simulink model "project"  (R2018b)
settings: Solver=FixedStepDiscrete  StartTime=0.0  StopTime=inf  FixedStep=3.1189083820662764e-10  RelTol=1e-3
values from neighbouring files (symbols this model uses):
  espacement_pilote = 4    [matlab.mat]
  N = 10    [matlab.mat]
  N_cyclic = 3    [matlab.mat]
  N_total = 16    [matlab.mat]
  Ts = 5.92592592593e-06    [matlab.mat]
undefined symbols (not defined in the file or in its folder): doppler
libraries: dspxfrm3 x5, commchan3 x2, commdigbbndpm3 x2, commrandsrc3 x1, commsink2 x1, dspfdesign x1
settings Model: SimulationMode=accelerator  Creator=rcalizzano  LastModifiedBy=nijac19
settings SolverCC: AutoInsertRateTranBlk=on
settings DataIOCC: LimitDataPoints=on  SaveOutput=off  SignalLogging=off  SaveTime=off
settings OptimizationCC: LifeSpan=inf
settings DebuggingCC: AlgebraicLoopMsg=error  SingleTaskRateTransMsg=error  AllowSymbolicDim=off  SFUnexpectedBacktrackingDiag=warning  SFNoUnconditionalDefaultTransitionDiag=warning  SFExecutionAtInitializationDiag=none
settings SFSimCC: SimUseLocalCustomCode=off
settings RTWCC: RTWUseLocalCustomCode=off
settings CodeAppCC: StateflowObjectComments=on
settings GRTTargetCC: TargetLangStandard=C89/C90 (ANSI)  GeneratePreprocessorConditionals=Disable all

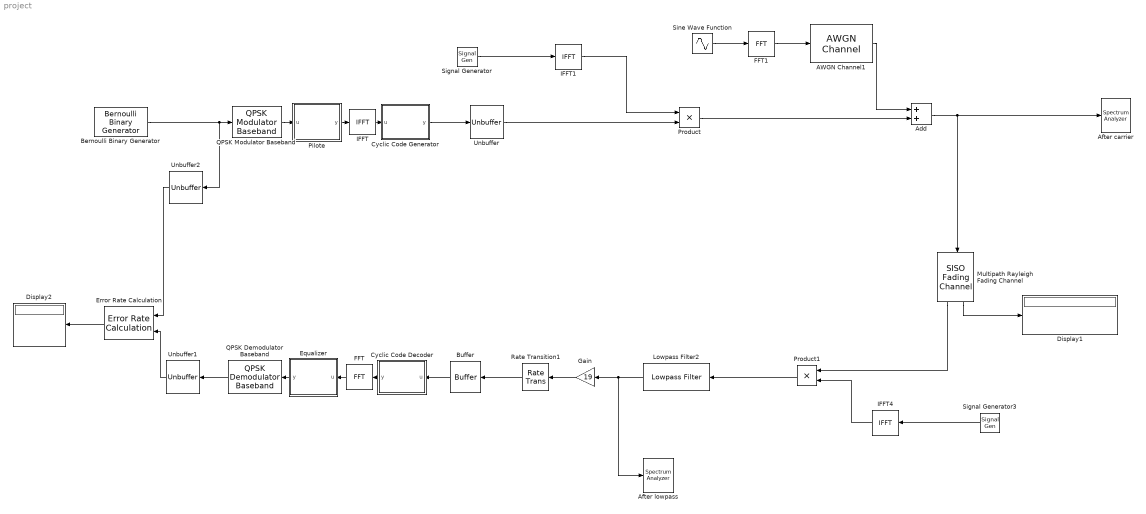
== system project ==
  AWGN Channel1 : commchan3/AWGN Channel  InputProcessing=Columns as channels (frame based)  seed=67  noiseMode="Signal to noise ratio  (SNR)"  EbNodB=10  EsNodB=10  SNRdB=150  bitsPerSym=1  Ps=4e4  Tsym=1  variance=1
  Add : Sum
  "After carrier " : SpectrumAnalyzer
  After lowpass : SpectrumAnalyzer
  Bernoulli Binary Generator : commrandsrc3/Bernoulli Binary Generator  ProbabilityOfZero=0.5  SeedSource=Auto  Seed=0  SampleTime=Ts/(N*2)  SamplesPerFrame=N*2  OutputDataType=double  SimulateUsing=Interpreted execution
      settings: SourceProductName=Communications Toolbox
  Buffer : Buffer  N=N_total+N_cyclic  OutputFrames=off
  Cyclic Code Decoder : MATLAB Function  TreatAsAtomicUnit=on
  Cyclic Code Generator : MATLAB Function  TreatAsAtomicUnit=on
  Display1 : Display
  Display2 : Display
  Equalizer : MATLAB Function  TreatAsAtomicUnit=on
  Error Rate Calculation : commsink2/Error Rate Calculation  N=N*2  st_delay=0  cp_mode=Entire frame  subframe=[]  PMode=Port  WsName=ErrorVec  RsMode2=off  stop=off  numErr=100  maxBits=1e6
      settings: SourceProductName=Communications Toolbox
  FFT : dspxfrm3/FFT  FFTImplementation=Auto  CompMethod=Table lookup  TableOpt=NEW  TableOptActive=Speed  BitRevOrder=off  Normalize=off  InheritFFTLength=on  FFTLength=64  WrapInput=on  roundingMode=Floor  overflowMode=off  firstCoeffDataTypeStr=Inherit: Same word length as input  firstCoeffLastDataTypeStr=Inherit: Same word length as input  outputMin=[]  outputMax=[]
  FFT1 : dspxfrm3/FFT  FFTImplementation=Auto  CompMethod=Table lookup  TableOpt=NEW  TableOptActive=Speed  BitRevOrder=off  Normalize=off  InheritFFTLength=on  FFTLength=64  WrapInput=on  roundingMode=Floor  overflowMode=off  firstCoeffDataTypeStr=Inherit: Same word length as input  firstCoeffLastDataTypeStr=Inherit: Same word length as input  outputMin=[]  outputMax=[]
  Gain : Gain  Gain=19
  IFFT : dspxfrm3/IFFT  FFTImplementation=Auto  CompMethod=Table lookup  TableOpt=NEW  TableOptActive=Speed  BitRevOrder=off  cs_in=off  Normalize=on  InheritFFTLength=on  FFTLength=64  WrapInput=on  mode=Complex  outSamplingMode=Sample based  roundingMode=Floor  overflowMode=off  firstCoeffDataTypeStr=Inherit: Same word length as input  firstCoeffLastDataTypeStr=Inherit: Same word length as input  outputMin=[]  outputMax=[]
      settings: SourceProductName=DSP System Toolbox
  IFFT1 : dspxfrm3/IFFT  FFTImplementation=Auto  CompMethod=Table lookup  TableOpt=NEW  TableOptActive=Speed  BitRevOrder=off  cs_in=off  Normalize=on  InheritFFTLength=on  FFTLength=64  WrapInput=on  mode=Complex  outSamplingMode=Sample based  roundingMode=Floor  overflowMode=off  firstCoeffDataTypeStr=Inherit: Same word length as input  firstCoeffLastDataTypeStr=Inherit: Same word length as input  outputMin=[]  outputMax=[]
      settings: SourceProductName=DSP System Toolbox
  IFFT4 : dspxfrm3/IFFT  FFTImplementation=Auto  CompMethod=Table lookup  TableOpt=NEW  TableOptActive=Speed  BitRevOrder=off  cs_in=off  Normalize=on  InheritFFTLength=on  FFTLength=64  WrapInput=on  mode=Complex  outSamplingMode=Sample based  roundingMode=Floor  overflowMode=off  firstCoeffDataTypeStr=Inherit: Same word length as input  firstCoeffLastDataTypeStr=Inherit: Same word length as input  outputMin=[]  outputMax=[]
      settings: SourceProductName=DSP System Toolbox
  Lowpass Filter2 : dspfdesign/Lowpass Filter  FilterType=IIR  DesignForMinimumOrder=on  FilterOrder=50  PassbandFrequency=fpass  StopbandFrequency=fstop  PassbandRipple=0.1  StopbandAttenuation=180  InheritSampleRate=on  SampleRate=1/15.5945e-009  SimulateUsing=Interpreted execution  roundingMode=Floor  coeffsDataTypeStr=fixdt(1,16)
  Multipath Rayleigh Fading Channel : commchan3/SISO Fading Channel  InheritSampleRate=on  SampleRate=1  PathDelays=[0]  AveragePathGains=[0]  NormalizePathGains=on  FadingDistribution=Rayleigh  KFactor=3  DirectPathDopplerShift=0  DirectPathInitialPhase=0  MaximumDopplerShift=0.01  DopplerSpectrum=doppler('Jakes')  ChannelInterpolationMethod=Polyphase  RandomStream=mt19937ar with seed  RandomNumGenerator=shr3cong  Seed=73  PathGainsOutputPort=on  ChannelFilterDelayOutputPort=off  SimulateUsing=Interpreted execution  Visualization=Off  PathsForDopplerDisplay=1  SamplesToDisplay=25%
      settings: SourceProductName=Communications Toolbox
  Pilote : MATLAB Function  TreatAsAtomicUnit=on
  Product : Product
  Product1 : Product
  QPSK Demodulator Baseband : commdigbbndpm3/QPSK Demodulator Baseband  OutType=Bit  DecType=Hard decision  VarSource=Dialog  Variance=1  Dec=Gray  Ph=pi/4  outDtype1=Inherit via internal rule  outDtype2=Inherit via internal rule  derotateFactorWordLen=16  derotateFactorDataTypeStr=Inherit: Same word length as input  derotateFactorLastDataTypeStr=Inherit: Same word length as input
      settings: SourceProductName=Communications Toolbox
  QPSK Modulator Baseband : commdigbbndpm3/QPSK Modulator Baseband  InType=Bit  Enc=Gray  Ph=pi/4  outDtype=double  outWordLen=16  outUDDataType=sfix(16)  outFracLenMode=Best precision  outFracLen=15  outDataTypeStr=double  outLastDataTypeStr=double
      settings: SourceProductName=Communications Toolbox
  Rate Transition1 : RateTransition
  Signal Generator : SignalGenerator  Amplitude=0.325  Frequency=868e6
  Signal Generator3 : SignalGenerator  Amplitude=0.325  Frequency=868e6
  Sine Wave Function : Sin  Amplitude=4e4  Frequency=314.159265  SampleTime=0
  Unbuffer : Unbuffer
  Unbuffer1 : Unbuffer
  Unbuffer2 : Unbuffer
  wires:
  QPSK Demodulator Baseband/1 -> Unbuffer1/1
  Unbuffer1/1 -> Error Rate Calculation/2
  Error Rate Calculation/1 -> Display2/1
  Unbuffer2/1 -> Error Rate Calculation/1
  Multipath Rayleigh Fading Channel/2 -> Display1/1
  Bernoulli Binary Generator/1 -> QPSK Modulator Baseband/1, Unbuffer2/1
  IFFT/1 -> Cyclic Code Generator/1(u)
  Cyclic Code Decoder/1(y) -> FFT/1
  QPSK Modulator Baseband/1 -> Pilote/1(u)
  Buffer/1 -> Cyclic Code Decoder/1(u)
  Equalizer/1(y) -> QPSK Demodulator Baseband/1
  Pilote/1(y) -> IFFT/1
  Cyclic Code Generator/1(y) -> Unbuffer/1
  FFT/1 -> Equalizer/1(u)
  IFFT1/1 -> Product/1
  Sine Wave Function/1 -> FFT1/1
  FFT1/1 -> AWGN Channel1/1
  Rate Transition1/1 -> Buffer/1
  AWGN Channel1/1 -> Add/1
  Product1/1 -> Lowpass Filter2/1
  Lowpass Filter2/1 -> After lowpass/1, Gain/1
  Signal Generator/1 -> IFFT1/1
  Gain/1 -> Rate Transition1/1
  Unbuffer/1 -> Product/2
  Signal Generator3/1 -> IFFT4/1
  IFFT4/1 -> Product1/2
  Product/1 -> Add/2
  Add/1 -> Multipath Rayleigh Fading Channel/1, "After carrier "/1
  Multipath Rayleigh Fading Channel/1 -> Product1/1

== matlab function project/Cyclic Code Decoder ==
  data: u input; y output; N_cyclic parameter
function y = fcn(u, N_cyclic)

y = u(N_cyclic+1:end);

== matlab function project/Pilote ==
  data: u input; N parameter; y output; N_total parameter; espacement_pilote parameter
function y  = fcn(u, N, N_total, espacement_pilote)

N_pilote = floor(N/espacement_pilote);
N_zeros = N_total-N-N_pilote;

w = complex(zeros(floor(N+N/espacement_pilote),1), zeros(floor(N+N/espacement_pilote),1));

% Insertion des pilotes

compteur = 0;
for i = [1:N]
    if mod(i,espacement_pilote) == espacement_pilote/2+1
        if compteur < N_pilote    
            w(i+compteur) = complex(1,0);
            compteur = compteur +1;
        end
        w(i+compteur) = u(i);
    else
        w(i+compteur) = u(i);
    end
end

% Insertion des zeros

y = [w(1:floor((N+floor(N/espacement_pilote))/2)); complex(zeros(N_zeros,1),zeros(N_zeros,1)); w(floor((N+floor(N/espacement_pilote))/2+1):end)];

== matlab function project/Cyclic Code Generator ==
  data: u input; y output; N_cyclic parameter; N_total parameter
function y = fcn(u, N_cyclic, N_total)

u_end = u(N_total-N_cyclic+1:end);

y = [u_end; u];

== matlab function project/Equalizer ==
  data: u input; y output; N parameter; N_total parameter; espacement_pilote parameter
function y = fcn(u, N, N_total, espacement_pilote)

N_pilote = floor(N/espacement_pilote);
N_zeros = N_total-N-N_pilote;

gain = complex(zeros(N_pilote,1), zeros(N_pilote,1));
gain_plot = complex(zeros(N_pilote+N,1), zeros(N_pilote+N,1));


% On enlève les zeros

w = [u(1:floor((N_total-N_zeros)/2)); u(floor((N_total-N_zeros)/2+N_zeros+1):end)];

% On initialise les valeurs des gains pour chaque sous canal

compteur_pilote = 1;

for i=[1:N+N_pilote]
    gain_plot(i) = 0;
    if mod(i,espacement_pilote+1) == espacement_pilote/2+1
        if compteur_pilote < N_pilote + 1
            gain(compteur_pilote) = w(i);
            gain_plot(i) = w(i);
            compteur_pilote = compteur_pilote+1;
        end
    end
end

gain_temp = ifft(gain);
gain_temporel = [gain_temp; complex(zeros(N,1), zeros(N,1))];
gain_total = fft(gain_temporel);
gain_final = [zeros(espacement_pilote/2,1)+gain_total(1); gain_total; zeros(espacement_pilote/2,1)+gain_total(N+N_pilote-espacement_pilote)];



% On égalise chaque sous canal

for i=[1:N_total-N_zeros]
   w(i) = w(i)/gain_final(i);
end

% On supprime les pilotes

y = [complex(zeros(N,1), zeros(N,1))];
compteur = 0;

for i=[1:N_total-N_zeros]
    if mod(i,espacement_pilote+1) == espacement_pilote/2+1
        if compteur > N_pilote - 1
            y(i-compteur)=w(i);
        else
            compteur = compteur + 1;
        end
    else
        y(i-compteur) = w(i);
    end
end
